simulink model "px4demo_uORBRead"  (R2019b)
settings: Solver=FixedStepAuto  StartTime=0.0  StopTime=inf  RelTol=1e-3  EnableMultiTasking=on
libraries: px4uORBlib x3
settings Model: SimulationMode=external  ExtModeTrigDuration=10  Creator=The MathWorks, Inc.  LastModifiedBy=The MathWorks, Inc.
settings SolverCC: PositivePriorityOrder=on
settings OptimizationCC: EnhancedBackFolding=on  PassReuseOutputArgsAs=Individual arguments  ZeroExternalMemoryAtStartup=off  ZeroInternalMemoryAtStartup=off  MaxStackSize=64  OptimizeBlockOrder=speed  DifferentSizesBufferReuse=on  OptimizationCustomize=off  EfficientTunableParamExpr=on
settings DebuggingCC: ParameterTunabilityLossMsg=error
settings HardwareCC: ProdBitPerPointer=32  ProdBitPerSizeT=32  ProdBitPerPtrDiffT=32  ProdLargestAtomicInteger=Long  ProdLargestAtomicFloat=Double  ProdWordSize=32  ProdLongLongMode=on  ProdHWDeviceType=ARM Compatible->ARM Cortex
settings SFSimCC: MATLABDynamicMemAlloc=off
settings RTWCC: SystemTargetFile=ert.tlc  HardwareBoard=PX4 Pixhawk 1  TLCOptions="-aInlineSetEventsForThisBaseRateFcn=TLC_FALSE -aSuppressMultiTaskScheduler=TLC_FALSE  -aRateBasedStepFcn=0"  TemplateMakefile=ert_default_tmf  GenerateReport=on  Toolchain=GNU Tools for PX4 Autopilots  IncludeHyperlinkInReport=on  LaunchReport=on  TargetLang=C++  GenerateTraceInfo=on  GenerateTraceReport=on  GenerateTraceReportSl=on  GenerateTraceReportSf=on  GenerateTraceReportEml=on
settings CodeAppCC: ForceParamTrailComments=on  IgnoreCustomStorageClasses=off  OperatorAnnotations=on  SimulinkDataObjDesc=on  SFDataObjDesc=on  InsertBlockDesc=on

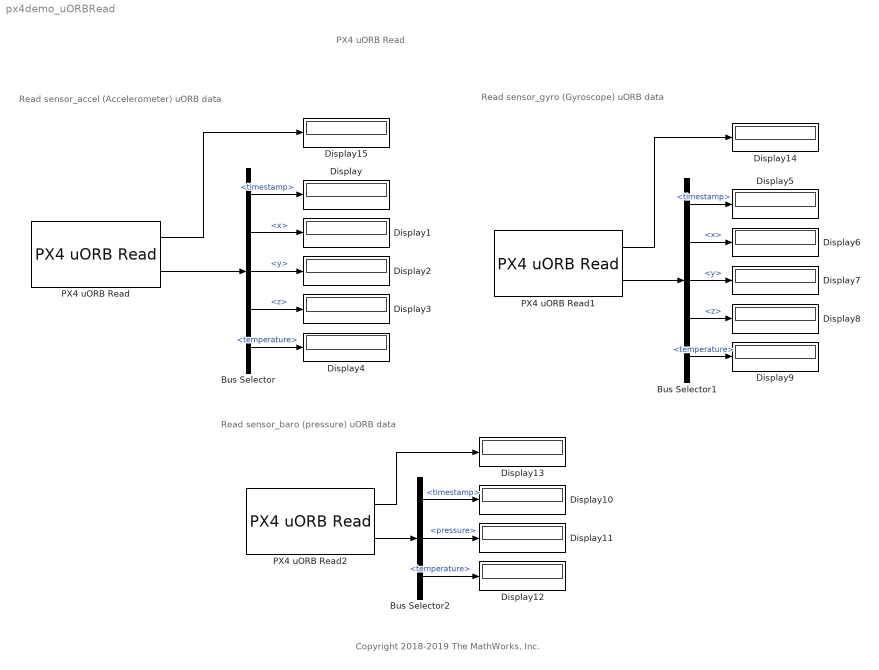
== system px4demo_uORBRead ==
  note: Copyright 2018-2019 The MathWorks, Inc.
  note: PX4 uORB Read
  note: Read sensor_accel (Accelerometer) uORB data
  note: Read sensor_gyro (Gyroscope) uORB data
  note: Read sensor_baro (pressure) uORB data
  Bus Selector : BusSelector  OutputSignals=timestamp,x,y,z,temperature
  Bus Selector1 : BusSelector  OutputSignals=timestamp,x,y,z,temperature
  Bus Selector2 : BusSelector  OutputSignals=timestamp,pressure,temperature
  Display{,1..15} (16 alike) : Display
  PX4 uORB Read : px4uORBlib/PX4 uORB Read  uORBTopic=sensor_accel  sampleTime=0.001  BlockingMode=off  BlockTimeout=1e-3
      settings: SourceProductName=Embedded Coder Support Package for PX4 Autopilots  SourceProductBaseCode=PX4AUTOPILOTS
  PX4 uORB Read1 : px4uORBlib/PX4 uORB Read  uORBTopic=sensor_gyro  sampleTime=0.01  BlockingMode=off  BlockTimeout=1e-3
      settings: SourceProductName=Embedded Coder Support Package for PX4 Autopilots  SourceProductBaseCode=PX4AUTOPILOTS
  PX4 uORB Read2 : px4uORBlib/PX4 uORB Read  uORBTopic=sensor_baro  sampleTime=1  BlockingMode=off  BlockTimeout=1e-3
      settings: SourceProductName=Embedded Coder Support Package for PX4 Autopilots  SourceProductBaseCode=PX4AUTOPILOTS
  wires:
  PX4 uORB Read/2 -> Bus Selector/1
  PX4 uORB Read1/2 -> Bus Selector1/1
  Bus Selector/1 -> Display/1  "<timestamp>"
  Bus Selector/2 -> Display1/1  "<x>"
  Bus Selector/3 -> Display2/1  "<y>"
  Bus Selector/4 -> Display3/1  "<z>"
  Bus Selector/5 -> Display4/1  "<temperature>"
  Bus Selector1/1 -> Display5/1  "<timestamp>"
  Bus Selector1/2 -> Display6/1  "<x>"
  Bus Selector1/3 -> Display7/1  "<y>"
  Bus Selector1/4 -> Display8/1  "<z>"
  Bus Selector1/5 -> Display9/1  "<temperature>"
  PX4 uORB Read2/2 -> Bus Selector2/1
  Bus Selector2/1 -> Display10/1  "<timestamp>"
  Bus Selector2/2 -> Display11/1  "<pressure>"
  Bus Selector2/3 -> Display12/1  "<temperature>"
  PX4 uORB Read2/1 -> Display13/1
  PX4 uORB Read1/1 -> Display14/1
  PX4 uORB Read/1 -> Display15/1
